simulink model "On_Off_Control"  (R2017b)
settings: Solver=VariableStepAuto  StartTime=0.0  StopTime=500  RelTol=1e-3  EnableMultiTasking=on
StartFcn:
  | clear all
libraries: realtime_pacer_lib x1
settings Model: Creator=johnh  LastModifiedBy=johnh
settings OptimizationCC: LifeSpan=inf
settings DebuggingCC: SFUnexpectedBacktrackingDiag=warning  SFNoUnconditionalDefaultTransitionDiag=warning  SFExecutionAtInitializationDiag=none
settings CodeAppCC: StateflowObjectComments=on
settings GRTTargetCC: TargetLangStandard=C89/C90 (ANSI)  GeneratePreprocessorConditionals=Disable all
settings ConfigComp: CovMetricSettings=dw  CovHtmlReporting=on  CovSaveCumulativeToWorkspaceVar=on  CovSaveSingleToWorkspaceVar=on  CovExternalEMLEnable=off

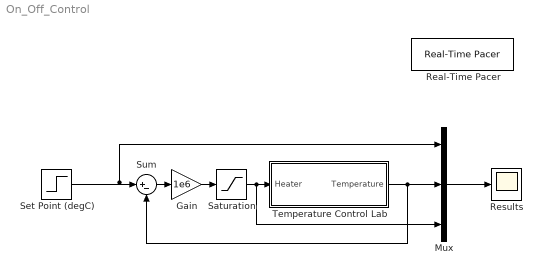
== system On_Off_Control ==
  Gain : Gain  Gain=1e6
  Mux : Mux  Inputs=3
  Real-Time Pacer : realtime_pacer_lib/Real-Time Pacer  simTimePerRealTime=1
  Results : Scope
  Saturation : Saturate  UpperLimit=100  LowerLimit=0
  Set Point (degC) : Step  Time=10  Before=25  After=35  SampleTime=0
  Sum : Sum  Inputs=|+-
  Temperature Control Lab : Subsystem
  wires:
  Temperature Control Lab/1(Temperature) -> Sum/2, Mux/2
  Set Point (degC)/1 -> Sum/1, Mux/1
  Mux/1 -> Results/1
  Saturation/1 -> Mux/3, Temperature Control Lab/1(Heater)
  Gain/1 -> Saturation/1
  Sum/1 -> Gain/1

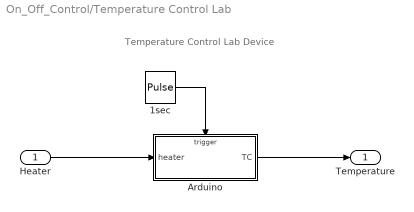
== system On_Off_Control/Temperature Control Lab ==
  note: Temperature Control Lab Device
  Heater : Inport
  1sec : DiscretePulseGenerator  PulseType=Time based  Period=1  PulseWidth=50
  Arduino : Subsystem  TreatAsAtomicUnit=on
  Temperature : Outport
  wires:
  1sec/1 -> Arduino/Trigger
  Arduino/1(TC) -> Temperature/1
  Heater/1 -> Arduino/1(heater)

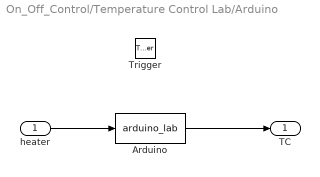
== system On_Off_Control/Temperature Control Lab/Arduino ==
  heater : Inport  LatchByDelayingOutsideSignal=on
  Trigger : TriggerPort  VariantControl=Variant
  Arduino : MATLABFcn  MATLABFcn=arduino_lab
  TC : Outport  InitialOutput=23
  wires:
  heater/1 -> Arduino/1
  Arduino/1 -> TC/1
